simulink model "simL0_multiPath"  (R2024a)
settings: Solver=ode4  StartTime=0.0  StopTime=1500  FixedStep=0.01  MaxStep=0.01  MinStep=10^-3  RelTol=0.01
values from neighbouring files (symbols this model uses):
  MegAWESkite = yaml.ReadYaml('MegAWESkite.yaml',false,true)    [runMain.m]
undefined symbols (not defined in the file or in its folder): actuatorLimit, controllerGains_retraction, controllerGains_traction, DiscIntNeverNeededParam, ENVMT, pathparam, simInit, tetherParams, winchParameter
libraries: simulink x9, slpidlib x9, sharedtransform x3, aerolibutil x3, dspswit3 x2, dspinverses x2, shared6dof x1, simulink_extras x1, dspsigops x1, dspstat3 x1, vrlib x1
(part 4 of 5)

== matlab function simL0_multiPath/Controls/ FlightControl/traction/Path_8_and_O ==
  data: target_p output; kite_posW input; c_i_prev input; closest_p output; s_cnew output; s_targ output; d_L1 output; dist_p output; pathparam parameter; c_i_prev output
% PATH-FOLLOWING-BLOCK_ FIGURE_OF_EIGHT 

%Description: This block implements the figure of eight path following
%             generating the desidered path in sphere as set of points 
%            
%             Determines the target point coordinates and closest point 
%             to the current aircraft position and both relative s value
%             on the path

function [target_p, closest_p, s_cnew, s_targ, d_L1, dist_p, c_i_prev] = ...
    path_wind_ref(kite_posW, c_i_prev, pathparam)

beta_el = pathparam.elevAng;
phi_az  = pathparam.polarAng;

k = pathparam.direction;
% negative: up loop or anti-clockwise 
% positive down loop or clockwise

R = sqrt(kite_posW(1).^2 + kite_posW(2).^2 + kite_posW(3).^2);

xc =  R * cos(beta_el)*cos(phi_az);      
yc =  R * cos(beta_el)*sin(phi_az);       %Center of the circle path
zc =  R * sin(beta_el);

pc = [xc, yc, zc];

% Define the normal vector to the plane aligned 
% with the vector btw center (ground station) and center of circle path
vc_n = pc/norm(pc); %down

% Choose two non-parallel vectors in the plane 
u = [-cos(beta_el)*cos(phi_az),cos(beta_el)*sin(phi_az),cos(beta_el)]; 

% Take the cross product of the two vectors to get a vector orthogonal to the plane 
v = cross(u, vc_n);

% NED basis for the plane
e1 = v / norm(u);   %E
e2 = u / norm(v);   %N
% e3 = -vc_n;       %D

% Define the range of s values
s = linspace(0,sign(k)*2*pi,50);           % (-) 2*pi to follow flight path in right direction

 %Generate the path [matrix coordinates]
r = pathparam.circRad;
abooth = pathparam.aBooth;
bbooth = pathparam.bBooth;
htau = pathparam.hTau;
if pathparam.isCircle
    % Function to generate circular pathshape
    [xP,yP,zP] = gen_circle(s, e1, e2, pc, R, r);
else
    % Function to generate Figure-of-eight pathshape
    [xP,yP,zP] = gen_path8(s, e1, e2, pc, R, abooth, bbooth, htau);
end

path = [xP;yP;zP];

%Calculates the distances from airc pos to every point on the path
d_to_p = sqrt((path(1,:) - kite_posW(1)).^2 + (path(2,:) - kite_posW(2)).^2 + (path(3,:) - kite_posW(3)).^2);

%Generate a circular vector of distances shifted in such a way that the
%first element
added_i = 5;
d_to_p_shift = circshift(d_to_p,-c_i_prev+added_i);  
d_to_p_shift = d_to_p_shift(1:25);            %Consider only 25 elems (half of the path)

[dist_p,i_d] = min(d_to_p_shift);      %Find index with minimum lenght

i_cnew = i_d + c_i_prev - added_i;       %Find the right index wrt s

if i_cnew <=0
    i_cnew = i_cnew + length(s);
end

if i_cnew >length(s)
   i_cnew = i_cnew - length(s);
end

c_i_prev = i_cnew;      %Update previuos closest index for next iteration
s_cnew = s(i_cnew);     %Calculates the corresponding s value of the index

%generate the closest point
if pathparam.isCircle
    [xC,yC,zC] = gen_circle(s_cnew, e1, e2, pc, R, r);
else
    [xC,yC,zC] = gen_path8(s_cnew, e1, e2, pc, R, abooth, bbooth, htau);
end
closest_p = [xC,yC,zC];

si = circshift(s,-c_i_prev);  

%Target point defined as np_head points wrt to closest point -> L1
s_targ = si(pathparam.numPoints_ahead);

%Generate the target point
if pathparam.isCircle
    [xT, yT, zT] = gen_circle(s_targ, e1, e2, pc, R, r);
else
    [xT, yT, zT] = gen_path8(s_targ, e1, e2, pc, R, abooth, bbooth, htau); 
end
target_p = [xT, yT, zT];

%Calculate the distance btw current aircraft pos and target point
d_L1 = sqrt((xT - kite_posW(1))^2 + (yT - kite_posW(2))^2 +(zT - kite_posW(3))^2);

end
 
function [xP,yP,zP] = gen_path8(s, e1, e2, pc, R, abooth, bbooth, htau)
    
    x_s = 1/htau * bbooth * sin(s) ./ (1 + (abooth/bbooth)^2 * cos(s).^2);
    y_s = 1/htau * abooth * sin(s) .* cos(s) ./ (1 + (abooth/bbooth)^2 * cos(s).^2);

    x = pc(1) + x_s * e1(1) + y_s * e2(1);
    y = pc(2) + x_s * e1(2) + y_s * e2(2);  % Path moved tangent to flight sphere
    z = pc(3) + x_s * e1(3) + y_s * e2(3);   

    xP = real(R * x./ sqrt(x.^2 + y.^2 + z.^2));
    yP = real(R * y./ sqrt(x.^2 + y.^2 + z.^2));  %Projection path on the sphere
    zP = real(R * z./ sqrt(x.^2 + y.^2 + z.^2));

end

function [xP,yP,zP] = gen_circle(s, e1, e2, pc, R, r)
% Parameters of circle path 
a=1;     %vertical component
b=1;     %orizontal component

%Path on the tangent plane in pc
x = pc(1) + a * r * (cos(s) * e2(1)) + b * r * (sin(s) * e1(1));
y = pc(2) + a * r * (cos(s) * e2(2)) + b * r * (sin(s) * e1(2));  
z = pc(3) + a * r * (cos(s) * e2(3)) + b * r * (sin(s) * e1(3));

%Projection path on the sphere
xP = real(R * x./ sqrt(x.^2 + y.^2 + z.^2));
yP = real(R * y./ sqrt(x.^2 + y.^2 + z.^2));  
zP = real(R * z./ sqrt(x.^2 + y.^2 + z.^2));
end

== matlab function simL0_multiPath/Controls/ FlightControl/Convert YPR-tantoe1 ==
  data: input input; roll output; pitch output; yaw output
%Function that convert Euler angles from actual tangential ref to earth

function [roll,pitch, yaw] = YPR_convert_tantoe(input)

%Aircraft position coordinates in earth ref system
x_a = input(1);
y_a = input(2);
z_a = input(3); 

[azi, el, r] = cart2sph(x_a,y_a,z_a); %Convert into spherical coordiantes
el = -el;            %Adjust to the definition positive elev angle pointing upwards
azi = -azi +pi/2;

%Aircraft euler rotation angles wrt to earth ref system
a_roll    = input(4);
a_pitch   = input(5);
a_yaw     = input(6);

%R_e = fromEuler(yaw, pitch, roll) -> define the rotation Rz*Ry*Rx
a_x = a_roll;
a_y = a_pitch;
a_z = a_yaw;

R = [cos(a_y)*cos(a_z), sin(a_x)*sin(a_y)*cos(a_z)-cos(a_x)*sin(a_z), cos(a_x)*sin(a_y)*cos(a_z)+sin(a_x)*sin(a_z);
     cos(a_y)*sin(a_z), sin(a_x)*sin(a_y)*sin(a_z)+cos(a_x)*cos(a_z), cos(a_x)*sin(a_y)*sin(a_z)-sin(a_x)*cos(a_z);
     -sin(a_y), sin(a_x)*cos(a_y), cos(a_x)*cos(a_y)];
 
%Building transformation matrix form eart to tan ref frame 
a_x = -el;
a_y = 0;
a_z = -azi;

R_1 = [cos(a_y)*cos(a_z), sin(a_x)*sin(a_y)*cos(a_z)-cos(a_x)*sin(a_z), cos(a_x)*sin(a_y)*cos(a_z)+sin(a_x)*sin(a_z);
     cos(a_y)*sin(a_z), sin(a_x)*sin(a_y)*sin(a_z)+cos(a_x)*cos(a_z), cos(a_x)*sin(a_y)*sin(a_z)-sin(a_x)*cos(a_z);
     -sin(a_y), sin(a_x)*cos(a_y), cos(a_x)*cos(a_y)];
 
a_x = 0;
a_y = pi/2;
a_z = -pi/2;  %Adjusted to obtain NED direction
 
R_2 = [cos(a_y)*cos(a_z), sin(a_x)*sin(a_y)*cos(a_z)-cos(a_x)*sin(a_z), cos(a_x)*sin(a_y)*cos(a_z)+sin(a_x)*sin(a_z);
     cos(a_y)*sin(a_z), sin(a_x)*sin(a_y)*sin(a_z)+cos(a_x)*cos(a_z), cos(a_x)*sin(a_y)*sin(a_z)-sin(a_x)*cos(a_z);
     -sin(a_y), sin(a_x)*cos(a_y), cos(a_x)*cos(a_y)];
 
R_etotan = R_1*R_2; %Earth to tan
R_tantoe = inv(R_etotan);

R_relativ=((R_tantoe)'*R);

%Extract euler Angles 
eul_l_p = zeros(1,3);
eul_l_p(2)=asin(-R_relativ(3,1));
if abs(eul_l_p(2)-pi/2)<1e-3
    eul_l_p(1)=0;
    eul_l_p(3)=atan2(R_relativ(2,3) - R_relativ(1,2),R_relativ(1,3)+R_relativ(2,2)+eul_l_p(1));
elseif abs(eul_l_p(2)+pi/2)<1e-3
    eul_l_p(1)=0;
    eul_l_p(3)=atan2(R_relativ(2,3) - R_relativ(1,2),R_relativ(1,3)+R_relativ(2,2)+eul_l_p(1));
else
    eul_l_p(1)=atan2(R_relativ(3,2),R_relativ(3,3));
    eul_l_p(3)=atan2(R_relativ(2,1),R_relativ(1,1));
end

roll = eul_l_p(1);                            
pitch = eul_l_p(2);  
yaw = eul_l_p(3);

end

== matlab function simL0_multiPath/Controls/ FlightControl/cart2spherical1 ==
  data: pos_aW input; r output; theta output; phi output
% Function to convert 3D Cartesian coordinates to spherical coordinates

function [r,theta,phi] = cart2spherical(pos_aW)

x = pos_aW(1);
y = pos_aW(2);
z = pos_aW(3);
% Calculate radial distance
r = sqrt(x.^2 + y.^2 + z.^2);

% Calculate polar angle
theta = atan2(y,x); % atan2 ensures the correct quadrant is chosen

% Calculate elevation angle
phi = asin(z./r); % acos returns values in [0,pi]

end

== matlab function simL0_multiPath/GroundStationMegAWES/Traction winch controller/Calculate Ft_ref/Zgraggen tether force reference ==
  data: v_ro input; Ft_ref output
function Ft_ref = fcn(v_ro)
% From Zgraggen (2016): "Automatic Retraction and Full-Cycle Operation for a
% Class of Airborne Wind Energy Generators".

C = 7.7008e3;  % Hard-coded for the MegAWES kite.
min_tetherf = 0.5e6;     %mention the choice of this values
max_tetherf = 1.0e6;

Ft_ref = 4*C*v_ro^2;

if v_ro <sqrt(min_tetherf/(4*C))
        Ft_ref = min_tetherf;
elseif v_ro > sqrt(max_tetherf/(4*C))
        Ft_ref = max_tetherf;
end

== matlab function simL0_multiPath/Environment_WindModel/MATLAB Function2 ==
  data: v_w_u input; v_w_p_mat output
% Copyright 2021 Delft University of Technology
%
% Licensed under the Apache License, Version 2.0 (the "License");
% you may not use this file except in compliance with the License.
% You may obtain a copy of the License at
%
%      http://www.apache.org/licenses/LICENSE-2.0
%
% Unless required by applicable law or agreed to in writing, software
% distributed under the License is distributed on an "AS IS" BASIS,
% WITHOUT WARRANTIES OR CONDITIONS OF ANY KIND, either express or implied.
% See the License for the specific language governing permissions and
% limitations under the License.

function v_w_p_mat = fcn(v_w_u)

v_w_p_mat = zeros( 3, length( v_w_u) );
v_w_p_mat(1,:) = v_w_u';

== matlab function simL0_multiPath/Controls/ FlightControl/Path_generation ==
  data: a_posW input; t_pointW output; s_cnew output; s_targ output; d_l1 output; dist_p output; pathparam parameter
function [t_pointW,s_cnew,s_targ,d_l1,dist_p]  = path(a_posW,pathparam)

persistent c_i_prev;
if isempty(c_i_prev)    %Index of the s vector to previous closest point
    c_i_prev = 30;      
end  

phi_el = pathparam.elevAng;
theta  = pathparam.polarAng;

k = pathparam.direction; 

R = sqrt(a_posW(1).^2 + a_posW(2).^2 + a_posW(3).^2);

xc =  R * cos(phi_el)*cos(theta);     
yc =  R * cos(phi_el)*sin(theta); 
zc =  R * sin(phi_el);

pc = [xc,yc,zc];    %center of the path

% Define the normal vector to the plane aligned 
% with the vector btw center (ground station) and center of circle path
vc = [xc,yc,zc];
vc_n = vc/norm(vc); %down

% Choose two non-parallel vectors in the plane 
u = [-cos(phi_el)*cos(theta),cos(phi_el)*sin(theta),sin(phi_el)]; 

% Take the cross product of the two vectors to get a vector orthogonal to the plane 
v = cross(u, vc_n);

% NED basis for the plane
e1 = v / norm(u);   %E
e2 = u / norm(v);   %N
e3 = -vc_n;          %D

s = linspace(0,k*2*pi,50);   % k defines the direction!!
r = pathparam.circRad;

function [xP,yP,zP] = gen_circle(s,e1,e2,pc,R,r)

% Parameters of circle path 
a=1;     %vertical component
b=1;     %orizontal component

%Path on the tangent plane in pc
x = pc(1) + a * r * (cos(s) * e2(1)) + b * r * (sin(s) * e1(1));
y = pc(2) + a * r * (cos(s) * e2(2)) + b * r * (sin(s) * e1(2));  
z = pc(3) + a * r * (cos(s) * e2(3)) + b * r * (sin(s) * e1(3));

%Projection path on the sphere
xP = real(R * x./ sqrt(x.^2 + y.^2 + z.^2));
yP = real(R * y./ sqrt(x.^2 + y.^2 + z.^2));  
zP = real(R * z./ sqrt(x.^2 + y.^2 + z.^2));

end

[xP,yP,zP] = gen_circle(s,e1,e2,pc,R,r);

path = [xP;yP;zP];  %Path matrix

%Vector of distances btw current pos and each point on the path
d_to_p = sqrt((path(1,:) - a_posW(1)).^2 + (path(2,:) - a_posW(2)).^2 + (path(3,:) - a_posW(3)).^2);

d_to_p_shift = circshift(d_to_p,-c_i_prev+5);   
d_to_p_shift = d_to_p_shift(1:25);

[dist_p,i_d] = min(d_to_p_shift); 
i_cnew = i_d + c_i_prev - 5; 

if i_cnew <=0
    i_cnew = i_cnew + length(s);
end
 
if i_cnew >length(s)
   i_cnew = i_cnew - length(s);
end

c_i_prev = i_cnew;  
s_cnew = s(i_cnew); 

[xC,yC,zC] = gen_circle(s_cnew,e1,e2,pc,R,r);  %generate the closest point
c_point = [xC,yC,zC];
si = circshift(s,-c_i_prev);  

 
s_targ = si(pathparam.np_ahead);   
[xT,yT,zT] = gen_circle(s_targ,e1,e2,pc,R,r);
t_pointW = [xT,yT,zT];

d_l1 = sqrt((xT - a_posW(1))^2 + (yT - a_posW(2))^2 +(zT - a_posW(3))^2);
%d_l1 = sqrt((xT - xC)^2 + (yT - yC)^2 +(zT - zC)^2);


end

== matlab function simL0_multiPath/Controls/ FlightControl/Heading_angle1 ==
  data: v_vel input; n output; v_targ input; v_tan output
% Function paht_tan_ang:

% It calculates the path angle on the tangential plane on the
% sphere knowing the projection on NE plane of the velocity (v_vel)
% and target (vector v)

function [n, v_tan]  = path_tan_ang(v_vel,v_targ)

%consider only the component on the NE plane
vec_vt = [v_vel(2) v_vel(3)];     %vector_velocity on tangential plane yz
vec_t = [v_targ(2) v_targ(3)];    %v_target


n = atan2(det([vec_vt; vec_t]), dot(vec_vt,vec_t));   
% the angle n is define btw velocity and target vector such as:
% + positive --> rotate vel clock-wise to reach target vect
% - negative --> rotate vel anti-clockwise to reach target vect

v_tan = sqrt(v_vel(2)*v_vel(2) +v_vel(3)*v_vel(3));

%Try another method to calculate the angle btw two vectors
% dot_product = dot(vec_vt, vec_t);
% 
% length_v = norm(vec_vt);
% length_t = norm(vec_t);
% 
% n1 = acos(dot_product / (length_v * length_t));

end

== matlab function simL0_multiPath/Controls/ FlightControl/traction/Tan_Transf matrix 1 ==
  data: cpos input; R_tantow output; R_wtorot output
% FUNCTION TRANSF_W2TAN

%This function defines all the transformation matrices from (W) wind frame
%to tangential plane on the current aircraft position on the sphere

% Input:  cpos current kite position in spherical coordinates (r,theta,phi)

% Output: R_tantow  Transformation matrix from tangential to wind ref frame
%         R_wtorot  Rotation matrix from wind to rotated (but centered) 
%                   tangential frame  (used to project velocities)

function [R_tantow, R_wtorot] = transf_w2tan(cpos)

r = cpos(1);
theta = cpos(2);
phi = cpos(3);


R_01 = [cos(theta) -sin(theta) 0 0; sin(theta) cos(theta) 0 0; 0 0 1 0; 0 0 0 1]; % matrice di rotazione attorno all'asse z
R_12 = [cos(phi) 0 -sin(phi) 0; 0 1 0 0; sin(phi) 0 cos(phi) 0; 0 0 0 1]; % matrice di rotazione attorno all'asse y
R_23 = [1 0 0 r; 0 1 0 0; 0 0 1 0; 0 0 0 1];
R_34 = [-1 0 0 0; 0 1 0 0; 0 0 1 0; 0 0 0 1];


R_rottow = R_01*R_12*R_34; %Rotation matrix between wind and oriented (non translated) sdf
R_wtorot = inv(R_rottow);

R_tantow = R_01 * R_12 * R_23* R_34; % Transf matrix from tangential to wind

end

== matlab function simL0_multiPath/Controls/ FlightControl/traction/cart2spherical1 ==
  data: pos_aW input; r output; theta output; phi output
% Function to convert 3D Cartesian coordinates to spherical coordinates

function [r,theta,phi] = cart2spherical(pos_aW)

x = pos_aW(1);
y = pos_aW(2);
z = pos_aW(3);
% Calculate radial distance
r = sqrt(x.^2 + y.^2 + z.^2);

% Calculate polar angle
theta = atan2(y,x); % atan2 ensures the correct quadrant is chosen

% Calculate elevation angle
phi = asin(z./r); % acos returns values in [0,pi]

end

== matlab function simL0_multiPath/Visualisation/Visualisation ==
  settings: updateMethod=DISCRETE  sampleTime=simInit.sample_time_vis
  data: t input; p_t_x input; p_t_y input; p_t_z input; pos_O input; eta_OB input; pathparam parameter; sampletime input; starget input
% Copyright 2021 Delft University of Technology
%
% Licensed under the Apache License, Version 2.0 (the "License");
% you may not use this file except in compliance with the License.
% You may obtain a copy of the License at
%
%      http://www.apache.org/licenses/LICENSE-2.0
%
% Unless required by applicable law or agreed to in writing, software
% distributed under the License is distributed on an "AS IS" BASIS,
% WITHOUT WARRANTIES OR CONDITIONS OF ANY KIND, either express or implied.
% See the License for the specific language governing permissions and
% limitations under the License.



%function Visualisation(t,p_t_x,p_t_y,p_t_z,Elevation, pos_O,eta_OB,params, sampletime) 
function Visualisation(t,p_t_x,p_t_y,p_t_z, pos_O,eta_OB, pathparam, sampletime, starget)   
    persistent handleTether
    persistent pathpoints
    persistent referencePath
    persistent Vert
    persistent handlePlane
    persistent targetPoint
    
    coder.extrinsic('plot3','patch','animatedline','addpoints');
 
    %% Figure settings
    if t==0
        figure(99)
%       addToolbarExplorationButtons(gcf)
        xlabel('x_W (m)');%, 'interpreter', 'latex')
        ylabel('y_W (m)');%, 'interpreter', 'latex')
        zlabel('z_W (m)');%, 'interpreter', 'latex')

        grid on
        box on;
        axis equal; hold on;

        view(30,21); % set the vieew angle for figure

        ax = [-500 1500];
        ay = [-1000 1000];
        az = [0 1200];
        axis([ax,ay,az]);  hold on

        X = [ax(1);ax(2);ax(2);ax(1)];
        Y = [ay(1);ay(1);ay(2);ay(2)];
        Z = [0;0;0;0];

        c = [0 1 0; % red
        0 1 0; % green
        0 1 0;
        0 1 0];
        fill3(X,Y,Z, c(:,2),'EdgeColor','none','FaceColor',c(1,:),'FaceAlpha',0.1);
    end
    
    %% Draw tether particles
    if isempty(handleTether)
 
        M_WO = [1, 0, 0; 
        0, -1, 0;
        0, 0, -1];
        pos_W = M_WO*[pos_O(1);pos_O(2);pos_O(3)];
        handleTether = plot3( [0;flipud(p_t_x);pos_W(1)], [0;flipud(p_t_y);pos_W(2)],[0;flipud(p_t_z);pos_W(3)],...
            '-', 'color', [0.1 0.1 0.1], 'Markersize',2, 'Linewidth', 1,...
            'MarkerFaceColor', [0.3 0.3 0.3]); hold on;
    end
    
    %% Draw aircraft
    if isempty(handlePlane)
        pn = pos_O(1);
        pe = pos_O(2);
        pd = pos_O(3);
        phi = eta_OB(1);
        theta = eta_OB(2);
        psi = eta_OB(3);
        
        M_WO = [1, 0, 0;  %original is [-1 0 0; 0 1 0; 0 0 -1] becouse winddir is pi/2
        0, -1, 0;
        0, 0, -1];
        
        scale = 10;
%         [F, Vert, C] = rndread('plane_thesis_big.stl');
        Image_kite = coder.load('plane_image.mat','F','Verti','C');
        F = Image_kite.F;
        Verti = Image_kite.Verti;
        C = Image_kite.C;
        Vert = scale*Verti'; 
        V = [ cos(psi)*cos(theta) , cos(psi)*sin(phi)*sin(theta) - cos(phi)*sin(psi) , sin(phi)*sin(psi) + cos(phi)*cos(psi)*sin(theta);
            cos(theta)*sin(psi)   , cos(phi)*cos(psi) + sin(phi)*sin(psi)*sin(theta) , cos(phi)*sin(psi)*sin(theta) - cos(psi)*sin(phi);
               -sin(theta)        ,             cos(theta)*sin(phi)                  ,             cos(phi)*cos(theta)                 ]...
               * Vert;
        V = V + [pn*ones(1,size(V,2));pe*ones(1,size(V,2));pd*ones(1,size(V,2))];
        V = M_WO*V;
        col =  [0, 0, 0];  %aircraft color black
        handlePlane = patch('faces', F, 'vertices' ,V');
        set(handlePlane, 'facec', 'k');              % Set the face color (force it)
        set(handlePlane, 'FaceVertexCData', C);       % Set the color (from file)
        set(handlePlane, 'EdgeColor','none');
        set(handlePlane, 'FaceLighting', 'none');
        set(handlePlane, 'FaceColor', col );
    end
    
    %% Draw black thin trail behind kite
    if isempty(pathpoints)
        pathpoints = animatedline('Linestyle','-','color', [1, 0, 0], 'Linewidth', .5);
    end
    
    %% Draw the target path in green
    if isempty(referencePath)
        phi_el = pathparam.elevAng;
        theta  = pathparam.polarAng;
        k=pathparam.direction;

        R = norm(pos_O);
        xc =  R * cos(phi_el)*cos(theta);     
        yc =  R * cos(phi_el)*sin(theta); 
        zc =  R * sin(phi_el);
        
        pc = [xc,yc,zc];
        
%         vc = [xc,yc,zc];
        vc_n = pc/norm(pc);
        u = [-cos(phi_el)*cos(theta),cos(phi_el)*sin(theta),sin(phi_el)]; 
        v = cross(u, vc_n);
        
        e1 = v / norm(u);   
        e2 = u / norm(v); 
        
        s = linspace(0,sign(k).*2*pi,100);  
        
        if pathparam.isCircle
            r = pathparam.circRad;
            [x,y,z] = gen_circle(s, e1, e2, pc, r);
        else
            aBooth = pathparam.aBooth;      
            bBooth = pathparam.bBooth;
            hTau   = pathparam.hTau; 
            [x,y,z] = gen_path8(s, e1, e2, pc, aBooth, bBooth, hTau);
        end

        xP = real(R * x./ sqrt(x.^2 + y.^2 + z.^2));
        yP = real(R * y./ sqrt(x.^2 + y.^2 + z.^2));  
        zP = real(R * z./ sqrt(x.^2 + y.^2 + z.^2));
        
        referencePath = plot3(xP,yP,zP, '-', 'color', [0 1 0],'Linewidth', 1.5);
        
        [~,i_targetPoint] = min(abs(abs(s)-abs(starget)));
        
        targetPoint = plot3(xP(i_targetPoint),yP(i_targetPoint),zP(i_targetPoint), 'x', 'color', [0 0 1],'MarkerSize', 20);
        
        plot3(pathparam.retractionTarget_W(1),pathparam.retractionTarget_W(2),pathparam.retractionTarget_W(3), 'x', 'color', [0 0 1],'MarkerSize', 10);
        
    end
        

% ------
    if (mod(t,sampletime)==0 && t~=0)
            %% Change each element on figure to current positions

            pn = pos_O(1);
            pe = pos_O(2);
            pd = pos_O(3);
            phi = eta_OB(1);
            theta = eta_OB(2);
            psi = eta_OB(3);

            M_WO = [1, 0, 0;    %original is [-1 0 0; 0 1 0; 0 0 -1] becouse winddir is pi/2
            0, -1, 0;
            0, 0, -1];

            % Tether
            set(handleTether,'XData',flipud(p_t_x), 'YData',flipud(p_t_y),'ZData',flipud(p_t_z));

            % Kite
            V = [ cos(psi)*cos(theta), cos(psi)*sin(phi)*sin(theta) - cos(phi)*sin(psi), sin(phi)*sin(psi) + cos(phi)*cos(psi)*sin(theta);
                cos(theta)*sin(psi), cos(phi)*cos(psi) + sin(phi)*sin(psi)*sin(theta), cos(phi)*sin(psi)*sin(theta) - cos(psi)*sin(phi);
                -sin(theta),                              cos(theta)*sin(phi),                              cos(phi)*cos(theta)] * Vert;
            V = V + [pn*ones(1,size(V,2));pe*ones(1,size(V,2));pd*ones(1,size(V,2))];
            V = M_WO*V;
            set(handlePlane, 'Vertices', V');

            % Trail
            pos_W = M_WO*[pn;pe;pd];
            addpoints(pathpoints,pos_W(1), pos_W(2),pos_W(3))
            %
            phi_el = pathparam.elevAng;
            theta  = pathparam.polarAng;
            k=pathparam.direction;

            R = norm(pos_O);
            xc =  R * cos(phi_el)*cos(theta);     
            yc =  R * cos(phi_el)*sin(theta); 
            zc =  R * sin(phi_el);

            pc = [xc,yc,zc];

            vc_n = pc/norm(pc);
            u = [-cos(phi_el)*cos(theta),cos(phi_el)*sin(theta),sin(phi_el)]; 
            v = cross(u, vc_n);

            e1 = v / norm(u);   
            e2 = u / norm(v); 
            
            s = linspace(0,sign(k).*2*pi,100);  

            if pathparam.isCircle
                r = pathparam.circRad;
                [x,y,z] = gen_circle(s, e1, e2, pc, r);
            else
                aBooth = pathparam.aBooth;      
                bBooth = pathparam.bBooth;
                hTau   = pathparam.hTau; 
                [x,y,z] = gen_path8(s, e1, e2, pc, aBooth, bBooth, hTau);
            end

            xP = real(R * x./ sqrt(x.^2 + y.^2 + z.^2));
            yP = real(R * y./ sqrt(x.^2 + y.^2 + z.^2));  
            zP = real(R * z./ sqrt(x.^2 + y.^2 + z.^2));

            set(referencePath,'XData',xP,'YData',yP,'ZData',zP);
            
             [~,i_targetPoint] = min(abs(abs(s)-abs(starget)));
             set(targetPoint,'XData',xP(i_targetPoint),'YData',yP(i_targetPoint),'ZData',zP(i_targetPoint));
        
    end
end

function [x,y,z] = gen_path8(s, e1, e2, pc, abooth, bbooth, htau)
    
    x_s = 1/htau .* bbooth .* sin(s) ./ (1 + (abooth/bbooth)^2 .* cos(s).^2);
    y_s = 1/htau.* abooth .* sin(s) .* cos(s) ./ (1 + (abooth/bbooth)^2 .* cos(s).^2);

    x = pc(1) + x_s .* e1(1) + y_s .* e2(1);
    y = pc(2) + x_s .* e1(2) + y_s .* e2(2);  % Path moved tangent to flight sphere
    z = pc(3) + x_s .* e1(3) + y_s .* e2(3);
end

function [x,y,z] = gen_circle(s, e1, e2, pc, r)
% Parameters of circle path 
a=1;     %vertical component
b=1;     %orizontal component

%Path on the tangent plane in pc
x = pc(1) + a .* r .* (cos(s) .* e2(1)) + b .* r .* (sin(s) .* e1(1));
y = pc(2) + a .* r .* (cos(s) .* e2(2)) + b .* r .* (sin(s) .* e1(2));  
z = pc(3) + a .* r .* (cos(s) .* e2(3)) + b .* r .* (sin(s) .* e1(3));
end

== matlab function simL0_multiPath/Computer 1/MATLAB Function ==
  data: s_path input; y output; s_old input; t input; t_old input; t_old output
function [y, t_old] = fcn(s_path, s_old, t, t_old)

    if (abs(s_path - s_old)>=9*pi/5) && t-t_old>=5
        y = true;
        t_old = t;
    else
        y = false;
    end
    
end

== matlab function simL0_multiPath/ParticleTetherModel/Tether_Dynamics ==
  data: kitePos input; tetherPos output; kiteVel input; windVel input; tetherLength input; x input; Ft_Ground output; Ft_Kite output; Fvec output; x output; ENVMT parameter; tetherParams parameter
% Copyright 2021 Delft University of Technology
%
% Licensed under the Apache License, Version 2.0 (the "License");
% you may not use this file except in compliance with the License.
% You may obtain a copy of the License at
%
%      http://www.apache.org/licenses/LICENSE-2.0
%
% Unless required by applicable law or agreed to in writing, software
% distributed under the License is distributed on an "AS IS" BASIS,
% WITHOUT WARRANTIES OR CONDITIONS OF ANY KIND, either express or implied.
% See the License for the specific language governing permissions and
% limitations under the License.

function [tetherPos, Ft_Ground, Ft_Kite, Fvec, x]= ...
    Tether_QuasiStatic(kitePos, kiteVel, windVel, tetherLength, x, ENVMT, tetherParams)
%#codegen

%Tether_QuasiStatic Trust-region dogleg nonlinear systems of equation
%   solver to determine the tether shape and forces.
%
%   Tether_QuasiStatic is based on the matlab implementation that 
%   solves a system of nonlinear equations using a dogleg
%   trust region approach.  The algorithm implemented is similar in nature
%   to the FORTRAN program HYBRD1 of J.J. More', B.S. Garbow and K.E. 
%   Hillstrom, User Guide for MINPACK 1, Argonne National Laboratory, 
%   Rept. ANL-80-74, 1980, which itself was based on the program CALFUN 
%   of M.J.D. Powell, A Fortran subroutine for solving systems of
%   nonlinear algebraic equations, Chap. 7 in P. Rabinowitz, ed.,
%   Numerical Methods for Nonlinear Algebraic Equations, Gordon and
%   Breach, New York, 1970.
%
%   Addapted by Ir. D. Eijkelhof (TU Delft) from 1990-2019 Matlab version 
%   The MathWorks, Inc.
% NOTE: From Matlab 2020b Matlab's Levenberg–Marquardt algorithm in the
% command "solve" can be directly used in codegen and might be
% faster. Due to availability of only matlab R2019B and lower, an own
% implementation had to be used in order the execute codegen.
%
% Syntax:  [tetherPos, Ft_Ground, Ft_Kite, Fvec, x]= ...
%     Tether_QuasiStatic(kitePos, kiteVel, windVel, tetherLength, x, ENVMT, T)
%
% NOTE: 'x' passed in and returned in column vector form.
%
% Throughout this routine 'x', 'F', 'xvec', 'xTrial', 'Fvec' and 'FTrial' are vectors.
%
% Inputs:
%    tetherPos  - Position vectors of tether particles
%    Ft_Ground  - Tether force magnitude at the ground station
%    Ft_Kite    - Tether force vector at the kite
%    Fvec       - Error between tether end and kite position (3D)
%    x          - Tether ground segment orientation and magnitude
%
% Outputs:
%    kitePos        - Kite position vector in wind reference frame
%    kiteVel        - Kite velocity vector in wind reference frame
%    windVel        - Wind velocity vector in wind reference frame
%    ENVMT          - Environmental parameters
%    tetherLength   - Reeled-out tether length determined by the winch
%    x              - Initial tether ground segment orientation and magnitude
%    tetherParams   - Tether dimensions and material properties
%
% Other m-files required: none
%
% Subfunctions: Objfunc    : Calculate difference between tether end and
%                            kite given tether ground segment orientation
%                            and magnitude.
%               testStop   : Test convergence criteria's
%               dogleg_tem : approximately solves trust region subproblem
%                            via a dogleg approach. 
%               lm_FD_J    : Determines the jacobian matrix by forward
%                            differencing
%
% MAT-files required: none
%
% Author: Dylan Eijkelhof, M.Sc.
% Delft University of Technology
% email address: d.eijkelhof@tudelft.nl  
% December 2019; Last revision: 16-March-2021

%------------- BEGIN CODE --------------
    
    [Fvec,T0,pj,~] = Objfunc(x,kitePos,kiteVel,windVel,tetherLength,ENVMT,tetherParams);
    
    xvec = x(:);         % vector representation of x
    % Convert values to full to avoid unnecessary sparse operation overhead
    % Initial x
    Fvec = full(Fvec); 
    
    % Set tolerances
    maxfunc     = 100*5;
    maxit       = 1000;
    tolf        = 1e-9;
    tolfunvalue = 1e-6;
    tolx        = 1e-6;
    tolobj      = 1e-6;
    
    nVar        = 3; % for codegen it worked better than numel(x)

    % Initialize local arrays.
    d           = zeros(nVar,1);

    % Initialize other trust region parameters.
    Delta       = 1e0;
    DeltaMax    = 1e10;
    eta1        = tetherParams.eta1;
    eta2        = tetherParams.eta2;
    alpha1      = tetherParams.alpha1;
    alpha2      = tetherParams.alpha2;

    % Extra initializations.
    iter        = 0;
    numFevals   = 1;

    stepAccept  = true;
    normd       = 0.0e0;
    objold      = 1.0e0;
    obj         = 0.5*(Fvec'*Fvec);  % Initial Fvec computed above

    numFDfevals = 0; %#ok<NASGU>
    JAC         = zeros(3,3); %#ok<PREALL> % pre-allocate derivative array

    %%%%%%%%%%%%%%%%%%%%%%% Calculate Jacobian at x0 %%%%%%%%%%%%%%%%%%
    [JAC,numFDfevals] = lm_FD_J(x, 0.1*ones(3,1),kitePos, kiteVel, ...
        windVel, tetherLength, ENVMT, tetherParams);

    % Increment the number of function evaluations with those used in the
    % finite difference calls.
    numFevals = numFevals + numFDfevals;

    grad = JAC'*Fvec;
    normgradinf = norm(grad,inf);

    % Test convergence at initial point.
    [done,~] = testStop(normgradinf,tolf,tolfunvalue,tolx,...
         stepAccept,iter,maxit,numFevals,maxfunc,Delta,normd,...
         obj,objold,d,xvec,tolobj,Fvec);

    % Beginning of main iteration loop.
    while ~done
    	iter = iter + 1;

    	% Compute step, d, using dogleg approach.
    	[d,quadObj,normd,normdscal] = ...
           dogleg(nVar,Fvec,JAC,grad,Delta);

        % Compute the model reduction given by d (pred).
        pred = -quadObj;

        % Compute the trial point, xTrial. Limit to positive value
        xTrial = xvec + d;
        if xTrial(3) < 0
            xTrial(3) = 1e-3;
        end

        % Evaluate nonlinear equations and objective at trial point.
        [F,T0,pj,~] = Objfunc(xTrial,kitePos,kiteVel,windVel,tetherLength,...
            ENVMT,tetherParams);
      
      
        numFevals = numFevals + 1;
        FTrial    = full(F(:)); % make FTrial a vector, convert to full
        objTrial  = 0.5*(FTrial'*FTrial); 

        % Compute the actual reduction given by xTrial (ared).
        ared      = obj - objTrial;

        % Compute ratio = ared/pred.
        if pred <= 0 % reject step
            ratio = 0;
        else
            ratio = ared/pred;
        end

        currTrialWellDefined = isfinite(objTrial);

        if ratio > eta1 && currTrialWellDefined % accept step.

            xvec    = xTrial; 
            objold  = obj; 
            obj     = objTrial;
            x(:)    = xvec; % update matrix representation
        
            %%%%%%%%%%%%%%%%%%%%%% Calculate New Jacobian %%%%%%%%%%%%%%%%%
            if iter == 1 || mod(iter,2*size(x,1))==0
                [JAC,numFDfevals] = lm_FD_J(x, 0.01*ones(3,1),kitePos, kiteVel, windVel, tetherLength, ENVMT, tetherParams);

                numFevals = numFevals + numFDfevals;
            else
                JAC = JAC + ((FTrial-Fvec-JAC*d)*d')/(d'*d);
            end
        
            Fvec        = FTrial; 
            grad        = JAC'*Fvec;
            normgradinf = norm(grad,inf);

            stepAccept  = true;
        else % reject step.
            stepAccept  = false;
        end 


        % Update trust region radius.
        if ~currTrialWellDefined
            % Shrink the trust region if any element of the function vector
            % at the new step is not defined (i.e. it's inf/NaN/complex). The
            % update for Delta in this case follows that in snls.
            Delta = min(normdscal/20,Delta/20);
        elseif ratio < eta1
            Delta = alpha2*normdscal;
        elseif ratio >= eta2
            Delta = max(Delta,alpha1*normdscal);
        end
        Delta = min(Delta,DeltaMax);

        % Check for termination.
        [done,~] = testStop(normgradinf,tolf,tolfunvalue,tolx,...
            stepAccept,iter,maxit,numFevals,maxfunc,Delta,normd,...
            obj,objold,d,xvec,tolobj,Fvec);
    end

    % Optimization is finished.  
    Ft_Ground   = x(3);
    Ft_Kite     = T0;
    tetherPos   = pj;
end

%%%%%%%%%%%%%%%%%%%%%%%%%%%%%%%%%%%%%%%%%%%%%%%%%%%%%%%%%%%%%%%
function [Fobj,T0,pj,p0] = Objfunc(stateVec,kitePos, kiteVel, windVel,...
                              tetherLength, ENVMT, tetherParams)
    Ns = size(windVel,2);       % number of masses
    Ls = tetherLength/(Ns+1);   % segment length
    mj = tetherParams.rho_t * Ls;          % segment mass

    p = kitePos;                % input aircraft position
    v = kiteVel;                % input aircraft velocity

    phi = stateVec(1);
    beta = stateVec(2);
    Tn = stateVec(3);

    omega_t = cross(p./(norm(p)^2),v);

    E = tetherParams.modulusE;
    A = tetherParams.A;

    FT = zeros(3,Ns); % Tension forces
    Fd = zeros(3,Ns); % Drag forces
    pj = zeros(3,Ns); % Mass positions
    vj = zeros(3,Ns); % Mass velocities
    aj = zeros(3,Ns); % Mass accellerations

    % First element from ground station (Ns)
    % FT(:,Ns) = Tn.*[sin(theta)* cos(phi); sin(phi); cos(theta)*cos(phi)];
    % pj(:,Ns) = Ls.*[sin(theta)* cos(phi); sin(phi); cos(theta)*cos(phi)];
    rotVec=[cos(phi)*cos(beta); sin(phi)*cos(beta); sin(beta)];
    FT(:,Ns) = Tn.*rotVec;
    pj(:,Ns) = Ls.*rotVec;
    vj(:,Ns) = dot(v,p./norm(p)) .* (p./norm(p)) + cross(omega_t,pj(:,Ns));
    aj(:,Ns) = cross(omega_t,cross(omega_t,pj(:,Ns)));
    
    % Drag calculation first element
    v_a_p = vj(:,Ns) - windVel(:,Ns);
    if all(abs(v_a_p)<1e-3)
        Fd(:,Ns) = [0;0;0];
    else
        v_a_p_t = dot((pj(:,Ns))/norm(pj(:,Ns)),v_a_p)*...
            ((pj(:,Ns))/norm(pj(:,Ns)));
        v_a_p_n = v_a_p - v_a_p_t;
        Fd(:,Ns) = -0.5 * ENVMT.rhos * Ls * tetherParams.d_tether * tetherParams.CD * ...
            norm(v_a_p_n) * v_a_p_n; % particle drag
    end
    
    % All other segments and masses except for segment connected to the kite
    for i = Ns:-1:2
        if i == Ns
            FT(:,i-1) = (mj+0.5*mj).*aj(:,i) + FT(:,i) - Fd(:,i) + ...
                [0;0;(mj+0.5*mj)*ENVMT.g];
        else
            FT(:,i-1) = mj.*aj(:,i) + FT(:,i) - Fd(:,i) + [0;0;mj*ENVMT.g];
        end

        l_i_1 = (norm(FT(:,i-1))/(E*A) + 1)*Ls;
        
        pj(:,i-1) = pj(:,i) + l_i_1.*(FT(:,i-1)/norm(FT(:,i-1)));       
        vj(:,i-1) = dot(v,p./norm(p)) .* (p./norm(p)) + cross(omega_t,pj(:,i-1));
        aj(:,i-1) = cross(omega_t,cross(omega_t,pj(:,i-1)));
        
        % Drag calculation
        v_a_p = vj(:,i) - windVel(:,i);
        if all(abs(v_a_p)<1e-3)
            Fd(:,i-1) = [0;0;0];
        else
            v_a_p_t = dot((pj(:,i-1)-pj(:,i))/norm(pj(:,i-1)-pj(:,i)),v_a_p) * ...
                ((pj(:,i-1)-pj(:,i))/norm(pj(:,i-1)-pj(:,i)));
            v_a_p_n = v_a_p - v_a_p_t;
            Fd(:,i-1) = -0.5 * ENVMT.rhos * Ls * tetherParams.d_tether * tetherParams.CD * ...
                norm(v_a_p_n) * v_a_p_n; % particle drag
        end
    end
    
    T0 = (mj+0.5*mj).*aj(:,1) + FT(:,1) - Fd(:,1) + [0;0;(mj+0.5*mj)*ENVMT.g];
    l_i_1 = (norm(T0)/(E*A) + 1)*Ls;
    p0 = pj(:,1) + l_i_1.*(T0/norm(T0));
    
    Fobj = p-p0;
end
%%%%%%%%%%%%%%%%%%%%%%%%%%%%%%%%%%%%%%%%%%%%%%%%%%%%%%%%%%%%%%%
function [done,EXITFLAG] = testStop(normgradinf,tolf,tolfunvalue,...
        tolx,stepAccept,iter,maxit,numFevals,maxfunc,Delta,normd,...
        obj,objold,d,xvec,tolobj,Fvec)
    %testStop checks the termination criteria for TRUSTNLEQN.

    done = false;
    EXITFLAG = 0;

    % Check termination criteria.

    if stepAccept && normgradinf < tolf
      EXITFLAG = 1;
      done = true;
      
    elseif iter > 1 && max(abs(d)./(abs(xvec)+1)) < max(tolx^2,eps)
       EXITFLAG = 2;
       done = true;
       
    elseif iter > 1 && stepAccept && normd < 0.9*Delta ...
                    && abs(objold-obj) < max(tolfunvalue^2,eps)*(1+abs(objold))
      EXITFLAG = 3;
      done = true;
      
    elseif iter > 1 && norm(Fvec) < tolobj
      EXITFLAG = 4;
      done = true;
      
    elseif Delta < 2*eps
      EXITFLAG = -3;
      done = true;
      
    elseif iter >= maxit
      EXITFLAG = 0;
      done = true;
      
    elseif numFevals >= maxfunc
      EXITFLAG = 0;
      done = true;
    end  
end
%%%%%%%%%%%%%%%%%%%%%%%%%%%%%%%%%%%%%%%%%%%%%%%%%%%%%%%%%%%%%%%
function [step,quadObj,normStep,normStepScal] = ...
    dogleg(nvar,F,JAC,grad,Delta)
%dogleg approximately solves trust region subproblem via a dogleg approach.
%
%   dogleg finds an approximate solution d to the problem:
%
%     min_d      f + g'd + 0.5*d'Bd
%
%     subject to ||Dd|| <= Delta
%
%   where g is the gradient of f, B is a Hessian approximation of f, D is a
%   diagonal scaling matrix and Delta is a given trust region radius.

%   Copyright 1990-2012 The MathWorks, Inc.
%   $Revision: 1.1.6.7 $  $Date: 2012/08/21 01:08:20 $

% NOTE: The scaling matrix D above is called scalMat in this routine.

% Compute scaled gradient and other scaled terms.
grad2 = grad;
normgradscal = norm(grad);

if normgradscal >= eps
    % First compute the Cauchy step (in scaled space).
    dCauchy = -(Delta/normgradscal)*grad;
    JACvec = JAC*grad2;
    denom = Delta*(JACvec'*JACvec);
    tauterm = normgradscal^3/denom;
    tauC = min(1,tauterm);
    dCauchy = tauC*dCauchy;
    
    % Compute quadratic objective at Cauchy point.
    JACvec = JAC*(dCauchy); 
    objCauchy = grad'*dCauchy + 0.5*(JACvec'*JACvec);   
    normdCauchy = min(norm(dCauchy),Delta);
else
    % Set Cauchy step to zero step and continue.
    objCauchy = 0;
    normdCauchy = 0;
    dCauchy = zeros(nvar,1);
end

if Delta - normdCauchy < eps
    % Take the Cauchy step if it is at the boundary of the trust region.
    step = dCauchy; quadObj = objCauchy;
else
    % Compute the Gauss-Newton step (in scaled space).
    
    dNewton = -JAC\F;
    
    if any(~isfinite(dNewton))
        % Take the Cauchy step if the Gauss-Newton step gives bad values.
        step = dCauchy; quadObj = objCauchy;
    else 
        normdNewt = norm(dNewton);
        if normdNewt <= Delta
            % Use the Newton direction as the trial step
            step = dNewton;
        else
            % Find the intersect point along dogleg path.
            Delta2 = Delta^2;
            normdCauchy2 = min(normdCauchy^2,Delta2);
            normdNewt2 = normdNewt^2;
            dCdN = dCauchy'*dNewton;
            dCdNdist2 = max((normdCauchy2+normdNewt2-2*dCdN),0);
            
            if dCdNdist2 == 0
                Lambda = 0;
            else
                % Stable method for solving 1-D quadratic
                a = 0.5*dCdNdist2;
                b = dCdN - normdCauchy2;
                c = 0.5*(normdCauchy2 - Delta2);
                q = -0.5*(b + sign(b)*sqrt(b^2 - 4*a*c));
                if b > 0
                    Lambda = c/q; 
                else
                    Lambda = q/a;
                end

                % Make sure we take a finite step,
                % (check for poorly scaled/infinite directions).
                if ~isfinite(Lambda)
                    Lambda = 0; % Take Cauchy step
                end
            end
            step = dCauchy + Lambda*(dNewton-dCauchy);
        end
        % Compute quadratic objective at trial point.
        JACvec = JAC*(step);
        quadObj = grad'*step + 0.5*(JACvec'*JACvec);
        
        % Compare Cauchy step and trial step (Newton or intersection)
        if objCauchy < quadObj
            step = dCauchy; quadObj = objCauchy;
        end
    end
end

% The step computed was the scaled step.  Unscale it.
normStepScal = norm(step);
normStep = norm(step);
end
 %%%%%%%%%%%%%%%%%%%%%%%%%%%%%%%%%%%%%%%%%%%%%%%%%%%%%%%%%%%%%%%
function [J,numFDfevals] = lm_FD_J(x, dp,kitePos, kiteVel, windVel, ...
                                tetherLength, ENVMT, tetherParams)

 m      = 3;                         % number of data points
 n      = 3;                         % number of parameters

 ps     = x; 
 J      = zeros(m,n); 
 del    = zeros(n,1);                % initialize Jacobian to Zero
 
 for j=1:n                           % START --- loop over all parameters

   del(j) = dp(j) * (1+abs(x(j)));   % parameter perturbation
   x(j)   = ps(j) + del(j);          % perturb parameter x(j)

   if del(j) ~= 0
     [y1,~,~,~] = Objfunc(x,kitePos, kiteVel, windVel, ...
         tetherLength, ENVMT, tetherParams);
     
     x(j) = ps(j) - del(j);
     [y,~,~,~] = Objfunc(x,kitePos, kiteVel, windVel, ...
         tetherLength, ENVMT, tetherParams);
     
     J(:,j) = (y1-y) ./ (2 .* del(j));
   end

   x(j) = ps(j);                     % restore x(j)

 end
 numFDfevals = 2;
                                     % END --- loop over all parameters
end

== matlab function simL0_multiPath/Output/MATLAB Function ==
  data: u input; y output
function y = fcn(u)

y = norm(u);

== matlab function simL0_multiPath/aerodynamic forces/Lookup Tables/Switch Solver Compiled ==
  data: input input double; out output double size=[10,1]; MegAWESkite parameter; ENVMT parameter; actuatorLimit parameter
%% switch sim after runtime

function out = simpleAero(input, MegAWESkite, ENVMT, actuatorLimit)
    coder.extrinsic('warning')

    % MAIN WING LOOK-UP TABLE
    alpha = atan2(input(3),input(1));
    beta = atan2(input(2),input(1));

%     alpha_damp = atan2((0.25*MegAWESkite.MainWing.MAC+MegAWESkite.cog(1))*input(5),...
%         input(1));
    alpha_damp=0;
    alpha_main = (MegAWESkite.MainWing.alpha0 + alpha+ alpha_damp)*180/pi;

    q = 0.5*ENVMT.rhos*input(1)^2;
    
    max_data_aoa = max(MegAWESkite.aero.mainwing.alpha);
    min_data_aoa = min(MegAWESkite.aero.mainwing.alpha);
    if alpha_main > max_data_aoa
        alpha_main = max_data_aoa;
    elseif alpha_main < min_data_aoa
        alpha_main = min_data_aoa;
    end
    
    alpha_aero = MegAWESkite.aero.mainwing.alpha;
    cl = MegAWESkite.aero.mainwing.main_cL;
    cd = MegAWESkite.aero.mainwing.main_cD;
    cm = MegAWESkite.aero.mainwing.main_cM;
    F_L_main = interp1(alpha_aero, cl, alpha_main,'spline') * q * ...
        MegAWESkite.MainWing.areaSurface;
    F_D_main = interp1(alpha_aero, cd, alpha_main,'spline') * q * ...
        MegAWESkite.MainWing.areaSurface;

%     F_x_mw = -F_D_main*cos(alpha)*cos(beta) + F_L_main*sin(alpha)*cos(beta);
    F_x_mw = -F_D_main*cos(alpha) + F_L_main*sin(alpha);
%     F_y_mw = -F_D_main*cos(alpha)*sin(beta) - F_L_main*sin(alpha)*sin(beta);
    F_y_mw = 0;
    F_z_mw = -F_L_main*cos(alpha);%+F_D_main*sin(alpha);

    act = sign(input(7))*max(abs(input(7)),abs(input(8)));
    maxAct = actuatorLimit.deflectionAileron;
    if act <= maxAct && act >= - maxAct
        c_roll_mw = act/maxAct * MegAWESkite.MainWing.main_max_c_Roll;
    elseif act > maxAct
        c_roll_mw = MegAWESkite.MainWing.main_max_c_Roll;
    else
        c_roll_mw = -MegAWESkite.MainWing.main_max_c_Roll;
    end
    
    M_x_mw = c_roll_mw * q * MegAWESkite.MainWing.areaSurface * ...
        MegAWESkite.MainWing.span;
    
    M_mw = interp1(alpha_aero, cm, alpha_main,'spline') * q * ...
        MegAWESkite.MainWing.areaSurface * MegAWESkite.MainWing.MAC;

    M_y_mw = M_mw - F_L_main*(0.25*MegAWESkite.MainWing.MAC+MegAWESkite.cog(1));

    out = [F_x_mw, F_y_mw, F_z_mw, M_x_mw, M_y_mw, 0, -F_L_main, alpha,0,0]';
end

== matlab function simL0_multiPath/Controls/ FlightControl/Retraction/Retraction heading ang ==
  data: kite_vel input; n output; kite_pos input; v_xy output; ang_vert output; ang_desired output; pathparam parameter; L1 output
% Function path angle for retraction phase
% Guidance law in earth ref frame

% velocity vector (vx,vy,vz) 
% target point (xt,yt,zt)



function [n, v_xy, ang_vert,ang_desired, L1] = path_ang(kite_vel,kite_pos,pathparam)  

target_point = pathparam.retractionTarget;
target_vector = target_point - kite_pos;

%consider only the component on the plane XY earth plane
v_xy = [kite_vel(1) kite_vel(2)];     
vec_t = [target_vector(1) target_vector(2)];   

%Calculate angle of vertical velocity wrt XY plane
ang_vert = -atan2(kite_vel(3), sqrt(kite_vel(1)^2 + kite_vel(2)^2));
ang_desired = -atan2(target_vector(3), sqrt(target_vector(1)^2 + target_vector(2)^2));

n = atan2(det([v_xy; vec_t]), dot(v_xy,vec_t));
L1 = norm(vec_t);

end

== matlab function simL0_multiPath/Controls/ FlightControl/Tan_Transf matrix 1 ==
  data: cpos input; R_tantow output; R_wtorot output
% FUNCTION TRANSF_W2TAN

%This function defines all the transformation matrices from (W) wind frame
%to tangential plane on the current aircraft position on the sphere

% Input:  cpos current kite position in spherical coordinates (r,theta,phi)

% Output: R_tantow  Transformation matrix from tangential to wind ref frame
%         R_wtorot  Rotation matrix from wind to rotated (but centered) 
%                   tangential frame  (used to project velocities)

function [R_tantow, R_wtorot] = transf_w2tan(cpos)

r = cpos(1);
theta = cpos(2);
phi = cpos(3);


R_01 = [cos(theta) -sin(theta) 0 0; sin(theta) cos(theta) 0 0; 0 0 1 0; 0 0 0 1]; % matrice di rotazione attorno all'asse z
R_12 = [cos(phi) 0 -sin(phi) 0; 0 1 0 0; sin(phi) 0 cos(phi) 0; 0 0 0 1]; % matrice di rotazione attorno all'asse y
R_23 = [1 0 0 r; 0 1 0 0; 0 0 1 0; 0 0 0 1];
R_34 = [-1 0 0 0; 0 1 0 0; 0 0 1 0; 0 0 0 1];


R_rottow = R_01*R_12*R_34; %Rotation matrix between wind and oriented (non translated) sdf
R_wtorot = inv(R_rottow);

R_tantow = R_01 * R_12 * R_23* R_34; % Transf matrix from tangential to wind

end

== matlab function simL0_multiPath/Controls/ FlightControl/Convert YPR-e_to_tan/Convert YPR-etotan ==
  data: input input; a_roll output; a_pitch output; a_yaw output
%Function that converts Euler angles from earth ref to tangential actual reference


function [a_roll,a_pitch, a_yaw] = YPR_convert_etotan(input)

%Aircraft position coordinates in earth ref system
x_a = input(1);
y_a = input(2);
z_a = input(3); 

[azi, el, r] = cart2sph(x_a,y_a,z_a); %Convert into spherical coordiantes
el = -el;            %Adjust to the definition positive elev angle pointing upwards
azi = -azi +pi/2;

%Aircraft euler rotation angles wrt to earth ref system
roll    = input(4);
pitch   = input(5);
yaw     = input(6);

%R_e = fromEuler(yaw, pitch, roll) -> define the rotation Rz*Ry*Rx
a_x = roll;
a_y = pitch;
a_z = yaw;

R = [cos(a_y)*cos(a_z), sin(a_x)*sin(a_y)*cos(a_z)-cos(a_x)*sin(a_z), cos(a_x)*sin(a_y)*cos(a_z)+sin(a_x)*sin(a_z);
     cos(a_y)*sin(a_z), sin(a_x)*sin(a_y)*sin(a_z)+cos(a_x)*cos(a_z), cos(a_x)*sin(a_y)*sin(a_z)-sin(a_x)*cos(a_z);
     -sin(a_y), sin(a_x)*cos(a_y), cos(a_x)*cos(a_y)];
 
%Building transformation matrix form eart to tan ref frame 
a_x = -el;
a_y = 0;
a_z = -azi;

R_1 = [cos(a_y)*cos(a_z), sin(a_x)*sin(a_y)*cos(a_z)-cos(a_x)*sin(a_z), cos(a_x)*sin(a_y)*cos(a_z)+sin(a_x)*sin(a_z);
     cos(a_y)*sin(a_z), sin(a_x)*sin(a_y)*sin(a_z)+cos(a_x)*cos(a_z), cos(a_x)*sin(a_y)*sin(a_z)-sin(a_x)*cos(a_z);
     -sin(a_y), sin(a_x)*cos(a_y), cos(a_x)*cos(a_y)];
 
a_x = 0;
a_y = pi/2;
a_z = -pi/2;  %Adjusted to obtain NED direction
 
R_2 = [cos(a_y)*cos(a_z), sin(a_x)*sin(a_y)*cos(a_z)-cos(a_x)*sin(a_z), cos(a_x)*sin(a_y)*cos(a_z)+sin(a_x)*sin(a_z);
     cos(a_y)*sin(a_z), sin(a_x)*sin(a_y)*sin(a_z)+cos(a_x)*cos(a_z), cos(a_x)*sin(a_y)*sin(a_z)-sin(a_x)*cos(a_z);
     -sin(a_y), sin(a_x)*cos(a_y), cos(a_x)*cos(a_y)];
 
R_etotan = R_1*R_2; %Earth to tan

R_relativ=((R_etotan)'*R);

%Extract euler Angles 
eul_l_p = zeros(1,3);
eul_l_p(2)=asin(-R_relativ(3,1));
if abs(eul_l_p(2)-pi/2)<1e-3
    eul_l_p(1)=0;
    eul_l_p(3)=atan2(R_relativ(2,3) - R_relativ(1,2),R_relativ(1,3)+R_relativ(2,2)+eul_l_p(1));
elseif abs(eul_l_p(2)+pi/2)<1e-3
    eul_l_p(1)=0;
    eul_l_p(3)=atan2(R_relativ(2,3) - R_relativ(1,2),R_relativ(1,3)+R_relativ(2,2)+eul_l_p(1));
else
    eul_l_p(1)=atan2(R_relativ(3,2),R_relativ(3,3));
    eul_l_p(3)=atan2(R_relativ(2,1),R_relativ(1,1));
end

a_roll = eul_l_p(1);                            
a_pitch = eul_l_p(2);  
a_yaw = eul_l_p(3);

end
